simulink model "Ejercicio13_16_02_17"  (R2013a)
settings: Solver=ode45  StartTime=0.0  StopTime=10  RelTol=1e-3
settings Model: Creator=Miguel  LastModifiedBy=Miguel

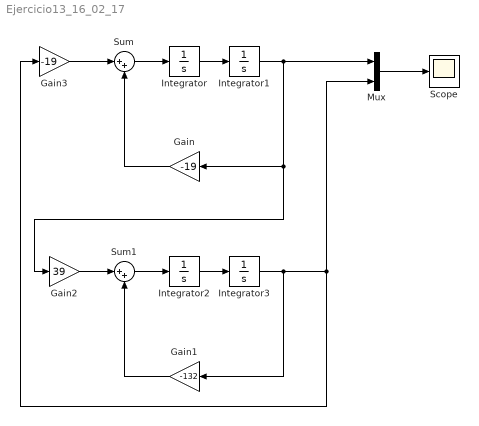
== system Ejercicio13_16_02_17 ==
  Gain : Gain  Gain=-19
  Gain1 : Gain  Gain=-132
  Gain2 : Gain  Gain=39
  Gain3 : Gain  Gain=-19
  Integrator : Integrator
  Integrator1 : Integrator  InitialCondition=10
  Integrator2 : Integrator
  Integrator3 : Integrator  InitialCondition=-5
  Mux : Mux  Inputs=2
  Scope : Scope
      settings: ShowLegends=on  TimeRange=10
  Sum : Sum  Inputs=|++
  Sum1 : Sum  Inputs=|++
  wires:
  Sum/1 -> Integrator/1
  Mux/1 -> Scope/1
  Integrator/1 -> Integrator1/1
  Gain/1 -> Sum/2
  Integrator1/1 -> Gain2/1, Gain/1, Mux/1
  Sum1/1 -> Integrator2/1
  Integrator2/1 -> Integrator3/1
  Gain1/1 -> Sum1/2
  Integrator3/1 -> Gain1/1, Gain3/1, Mux/2
  Gain2/1 -> Sum1/1
  Gain3/1 -> Sum/1
